simulink model "CACC"  (R2020a)
settings: Solver=VariableStepAuto  StartTime=0.0  StopTime=100  RelTol=1e-3
InitFcn:
  | totalVehicles = 2;
  | if exist('vehStatesBus', 'var')==0
  | load vehBuses
  | end
  | if exist('vehErrorsBus', 'var')==0
  | load vehBuses
  | end
libraries: simulink x9, sim3dlib x2, sim3dautolib x2, autolibshared x2, visionsinks x1
settings Model: Creator=fvall  LastModifiedBy=fvall

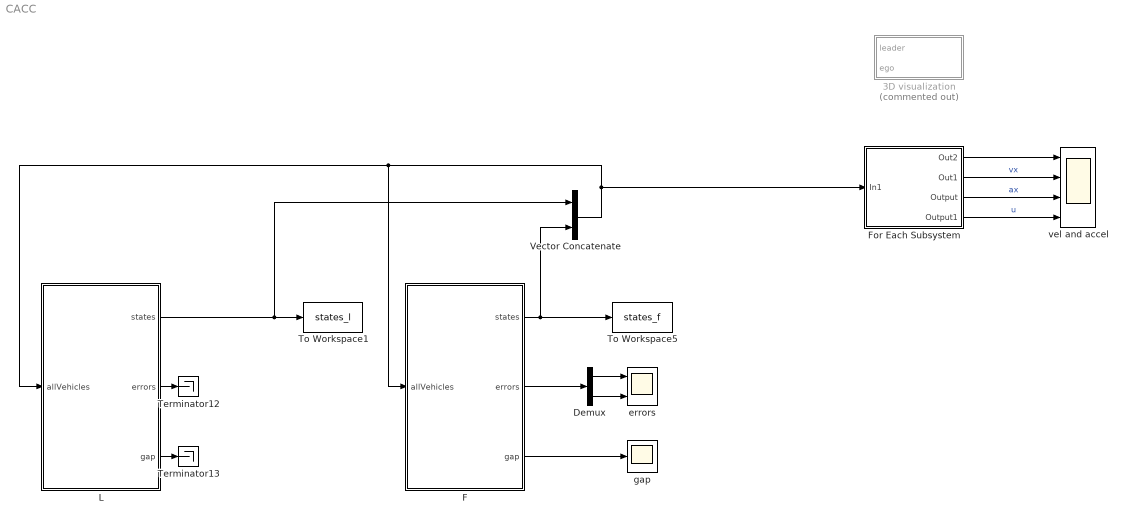
== system CACC ==
  3D visualization : Subsystem  Commented=on
  Demux : Demux  Outputs=2
  F : Subsystem  mask{m=2000, lf=2.5, lr=2.5, maxAcceleration=3, minAcceleration=-8, maxJerk=50, minJerk=-50, freeFlowVel=25, tau=0.5, x0=0, vx0=20, y0=0, h=0.56375, d0=0.32452, minHeadwayError=-100, maxHeadwayError=Inf, velFilterGain=10, Kd=1.7738, Kp=0.17738, Ki=0, Ka=0.97561, Kdd=0.097561, velKi=0.0019848, velKp=0.052702, velKd=-0.65465, hFilterGain=1, hFilterSaturation=0.5, vMin=13, maxComfAccel=0.6, minComfAccel=-0.4, maxComfJerk=10, minComfJerk=-10, hLC=1.6381, d0LC=0.32452}
      mask prompts: m "autoblks_shared:autoblkVehBody3DofLat:blkPrm_m"; lf "autoblks_shared:autoblkVehBody3DofLat:blkPrm_a"; lr "autoblks_shared:autoblkVehBody3DofLat:blkPrm_b"; maxAcceleration "Max Acceleration"; minAcceleration "Min Acceleration"; maxJerk "Max Jerk"; minJerk "Min Jerk"; freeFlowVel "Free Flow Velocity"; tau "Actuator Lag"; x0 "autoblks_shared:autoblkVehBody3DofLat:blkPrm_X_o"; vx0 "autoblks_shared:autoblkVehBody3DofLat:blkPrm_xdot_o"; y0 "autoblks_shared:autoblkVehBody3DofLat:blkPrm_Y_o"; h "Time Headway"; d0 "Standstill Gap"; minHeadwayError "Min Headway Error"; maxHeadwayError "Max Headway Error"; velFilterGain "Velocity Filter Gain"; hFilterGain "Headway Filter Gain"; hFilterSaturation "Headway Filter Saturation"; vMin "Min Velocity"; maxComfAccel "Max Comf Accel"; minComfAccel "Min Comf Accel"; maxComfJerk "Max Comf Jerk"; minComfJerk "Min Comf Jerk"; hLC "Time Headway LC"; d0LC "Standstill Gap LC"
      mask TypeOptions m: Vehicle Body 3DOF Single Track/m
      mask TypeOptions lf: Vehicle Body 3DOF Single Track/a
      mask TypeOptions lr: Vehicle Body 3DOF Single Track/b
      mask TypeOptions x0: Vehicle Body 3DOF Single Track/X_o
      mask TypeOptions vx0: Vehicle Body 3DOF Single Track/xdot_o
      mask TypeOptions y0: Vehicle Body 3DOF Single Track/Y_o
      mask DialogControl DescGroupVar Prompt: 3DOF Vehicle with ACC
      mask DialogControl DescTextVar Prompt: Vehicle with ACC. The vehicle model is Simulink's 3DOF single track vehicle body. The controller is a PID with constant headway including headway error saturation and filtered leader velocity.
      mask DialogControl VehParams Prompt: Vehicle Parameters
      mask DialogControl m Prompt: Vehicle mass, m [kg]:
      mask DialogControl lf Prompt: Longitudinal distance from center of mass to front axle, a [m]:
      mask DialogControl lr Prompt: Longitudinal distance from center of mass to rear axle, b [m]:
      mask DialogControl InitStates Prompt: Initial State
      mask DialogControl x0 Prompt: Initial inertial frame longitudinal position, X_o [m]:
      mask DialogControl vx0 Prompt: Initial longitudinal velocity, xdot_o [m/s]:
      mask DialogControl y0 Prompt: Initial inertial frame lateral displacement, Y_o [m]:
      mask DialogControl Container3 Prompt: Veh Following Parameters
      mask DialogControl ComfortConstraints Prompt: Comfort Constraints
      mask DialogControl LaneChangeParams Prompt: Lane Change Params
  For Each Subsystem : Subsystem  TreatAsAtomicUnit=on
  L : Subsystem  mask{m=2000, lf=2.5, lr=2.5, maxAcceleration=3, minAcceleration=-8, maxJerk=50, minJerk=-50, freeFlowVel=20, tau=0.5, x0=316.5995, vx0=20, y0=0, h=0.56375, d0=0.32452, minHeadwayError=-100, maxHeadwayError=Inf, velFilterGain=10, Kd=1.7738, Kp=0.17738, Ki=0, Ka=0.97561, Kdd=0.097561, velKi=0.0019848, velKp=0.052702, velKd=-0.65465, hFilterGain=1, hFilterSaturation=0.5, vMin=13, maxComfAccel=0.6, minComfAccel=-0.4, maxComfJerk=10, minComfJerk=-10, hLC=1.6381, d0LC=0.32452}
      mask prompts: m "autoblks_shared:autoblkVehBody3DofLat:blkPrm_m"; lf "autoblks_shared:autoblkVehBody3DofLat:blkPrm_a"; lr "autoblks_shared:autoblkVehBody3DofLat:blkPrm_b"; maxAcceleration "Max Acceleration"; minAcceleration "Min Acceleration"; maxJerk "Max Jerk"; minJerk "Min Jerk"; freeFlowVel "Free Flow Velocity"; tau "Actuator Lag"; x0 "autoblks_shared:autoblkVehBody3DofLat:blkPrm_X_o"; vx0 "autoblks_shared:autoblkVehBody3DofLat:blkPrm_xdot_o"; y0 "autoblks_shared:autoblkVehBody3DofLat:blkPrm_Y_o"; h "Time Headway"; d0 "Standstill Gap"; minHeadwayError "Min Headway Error"; maxHeadwayError "Max Headway Error"; velFilterGain "Velocity Filter Gain"; hFilterGain "Headway Filter Gain"; hFilterSaturation "Headway Filter Saturation"; vMin "Min Velocity"; maxComfAccel "Max Comf Accel"; minComfAccel "Min Comf Accel"; maxComfJerk "Max Comf Jerk"; minComfJerk "Min Comf Jerk"; hLC "Time Headway LC"; d0LC "Standstill Gap LC"
      mask TypeOptions m: Vehicle Body 3DOF Single Track/m
      mask TypeOptions lf: Vehicle Body 3DOF Single Track/a
      mask TypeOptions lr: Vehicle Body 3DOF Single Track/b
      mask TypeOptions x0: Vehicle Body 3DOF Single Track/X_o
      mask TypeOptions vx0: Vehicle Body 3DOF Single Track/xdot_o
      mask TypeOptions y0: Vehicle Body 3DOF Single Track/Y_o
      mask DialogControl DescGroupVar Prompt: 3DOF Vehicle with ACC
      mask DialogControl DescTextVar Prompt: Vehicle with ACC. The vehicle model is Simulink's 3DOF single track vehicle body. The controller is a PID with constant headway including headway error saturation and filtered leader velocity.
      mask DialogControl VehParams Prompt: Vehicle Parameters
      mask DialogControl m Prompt: Vehicle mass, m [kg]:
      mask DialogControl lf Prompt: Longitudinal distance from center of mass to front axle, a [m]:
      mask DialogControl lr Prompt: Longitudinal distance from center of mass to rear axle, b [m]:
      mask DialogControl InitStates Prompt: Initial State
      mask DialogControl x0 Prompt: Initial inertial frame longitudinal position, X_o [m]:
      mask DialogControl vx0 Prompt: Initial longitudinal velocity, xdot_o [m/s]:
      mask DialogControl y0 Prompt: Initial inertial frame lateral displacement, Y_o [m]:
      mask DialogControl Container3 Prompt: Veh Following Parameters
      mask DialogControl ComfortConstraints Prompt: Comfort Constraints
      mask DialogControl LaneChangeParams Prompt: Lane Change Params
  Terminator12 : Terminator
  Terminator13 : Terminator
  To Workspace1 : ToWorkspace  VariableName=states_l  SaveFormat=Timeseries  SampleTime=-1
  To Workspace5 : ToWorkspace  VariableName=states_f  SaveFormat=Timeseries  SampleTime=-1
  Vector Concatenate : Concatenate
  errors : Scope  NumInputPorts=2
  gap : Scope
  vel and accel : Scope  NumInputPorts=4
  wires:
  L/1(states) -> Vector Concatenate/1, To Workspace1/1
  F/1(states) -> To Workspace5/1, Vector Concatenate/2
  Vector Concatenate/1 -> F/1(allVehicles), L/1(allVehicles), For Each Subsystem/1(In1)
  F/2(errors) -> Demux/1
  Demux/1 -> errors/1
  Demux/2 -> errors/2
  F/3(gap) -> gap/1
  For Each Subsystem/3(Output) -> vel and accel/3  "ax"
  For Each Subsystem/2(Out1) -> vel and accel/2  "vx"
  L/2(errors) -> Terminator12/1
  L/3(gap) -> Terminator13/1
  For Each Subsystem/4(Output1) -> vel and accel/4  "u"
  For Each Subsystem/1(Out2) -> vel and accel/1

== system CACC/3D visualization ==
  leader : Inport
  ego : Inport  Port=2
  Bus Selector : BusSelector  OutputSignals=InertFrm.Geom.Disp.X,InertFrm.Geom.Disp.Y,InertFrm.Cg.Ang.psi
  Bus Selector1 : BusSelector  OutputSignals=InertFrm.Geom.Disp.X,InertFrm.Geom.Disp.Y,InertFrm.Cg.Ang.psi
  Simulation 3D Camera Get : sim3dlib/Simulation 3D Camera Get  Priority=1  sensorTag=Sim3dSensor1  sensorId=1  sensorName=Sim3dSensor1  vehTagList={'Scene Origin';'SimulinkVehicle1';'SimulinkVehicle2'}  vehTag=SimulinkVehicle1  mountLoc=Rearview mirror  offsetFlag=off  tmountOffset=[0, 0, 0]  rmountOffset=[0, 0, 0]  HorizontalResolution=1280  VerticalResolution=720  HorizontalFOV=60  SampleTime=-1  mountPoint=[0.319999992847443 0 1.19000005722046]  mountOrientation=[0 0 0]  aMode=2  ID=1
      settings: SourceProductBaseCode=DR,VE
  Simulation 3D Scene Configuration : sim3dlib/Simulation 3D Scene Configuration  Priority=0  ProjectFormat=Default Scenes  SceneDesc=Straight road  ProjectName=VehicleSimulation.exe  ScenePath=/Game/Maps/HwStrght  vehTagList={'Scene Origin';'SimulinkVehicle1'}  vehTag=SimulinkVehicle1  OpVisEn=off  Ts=1/60  EnableWindow=on  sensorTag=MainCamera1  sensorId=1  sensorName=MainCamera1  mountLoc=Origin  offsetFlag=off  tmountOffset=[0, 0, 0]  rmountOffset=[0, 0, 0]  HorizontalResolution=1280  VerticalResolution=720  HorizontalFOV=60  mountPoint=[0 0 0]  mountOrientation=[0 0 0]  aMode=3  ID=1
      settings: SourceProductBaseCode=DR,VE
  Simulation 3D Vehicle with Ground Following : sim3dautolib/Simulation 3D Vehicle with Ground Following  Priority=-1  PassVehMesh=Muscle car  VehColor=Red  InitialPos=[0, 0, 0]  InitialRot=[0, 0, 0]  ActorName=SimulinkVehicle1  SampleTime=-1  ActorType=SimulinkVehicle  ID=1  aMode=3  ActorTag=SimulinkVehicle1  CoordinateScheme=ISO  TransformOutportEnabled=off
      settings: SourceProductBaseCode=DR,VE
  Simulation 3D Vehicle with Ground Following1 : sim3dautolib/Simulation 3D Vehicle with Ground Following  Priority=-1  PassVehMesh=Muscle car  VehColor=Red  InitialPos=[0, 0, 0]  InitialRot=[0, 0, 0]  ActorName=SimulinkVehicle2  SampleTime=-1  ActorType=SimulinkVehicle  ID=2  aMode=3  ActorTag=SimulinkVehicle2  CoordinateScheme=ISO  TransformOutportEnabled=off
      settings: SourceProductBaseCode=DR,VE
  Unit Conversion : UnitConversion
  Unit Conversion1 : UnitConversion
  Video To Workspace : visionsinks/Video To Workspace  VariableName=vout  NumInputs=1  DataLimit=1000  DecimationFactor=1  LogFi=off  InPortLabels=R|G|B
      settings: SourceProductBaseCode=VP
  wires:
  Unit Conversion/1 -> Simulation 3D Vehicle with Ground Following/3
  ego/1 -> Bus Selector/1
  Bus Selector/1 -> Simulation 3D Vehicle with Ground Following/1  "<X>"
  Bus Selector/2 -> Simulation 3D Vehicle with Ground Following/2  "<Y>"
  Bus Selector/3 -> Unit Conversion/1  "<psi>"
  Unit Conversion1/1 -> Simulation 3D Vehicle with Ground Following1/3
  leader/1 -> Bus Selector1/1
  Bus Selector1/1 -> Simulation 3D Vehicle with Ground Following1/1  "<X>"
  Bus Selector1/2 -> Simulation 3D Vehicle with Ground Following1/2  "<Y>"
  Bus Selector1/3 -> Unit Conversion1/1  "<psi>"
  Simulation 3D Camera Get/1 -> Video To Workspace/1

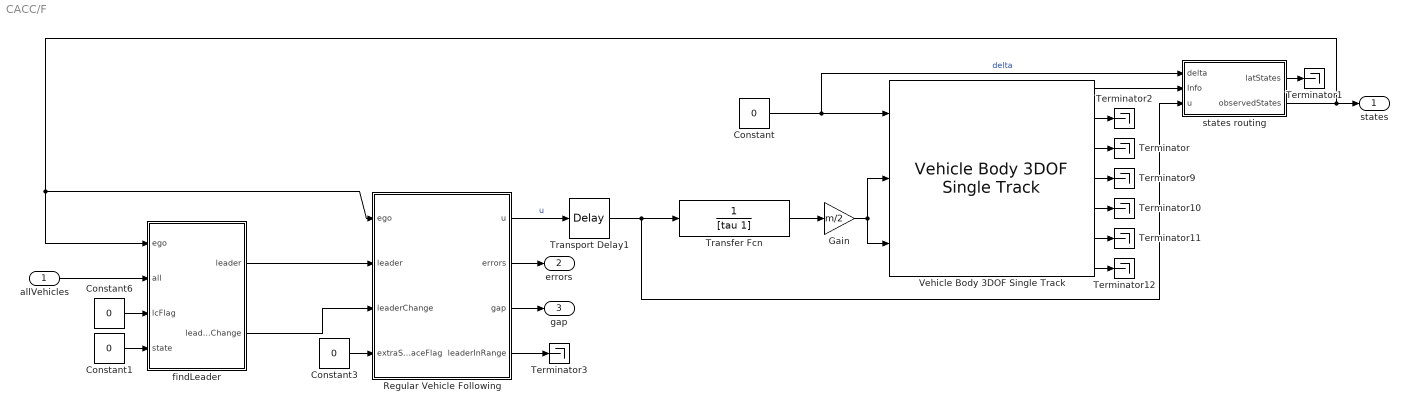
== system CACC/F ==
  allVehicles : Inport
  Constant{,1,3,6} (4 alike) : Constant  Value=0
  Gain : Gain  Gain=m/2
  Regular Vehicle Following : Subsystem
  Terminator{,1..3,9..12} (8 alike) : Terminator
  Transfer Fcn : TransferFcn  Denominator=[tau 1]
  Transport Delay1 : TransportDelay  DelayTime=0.01
  Vehicle Body 3DOF Single Track : autolibshared/Vehicle Body 3DOF Single Track  trackMode=Single (bicycle)  inputMode=External longitudinal forces  frontSteerMode=on  rearSteerMode=off  windMode=off  muMode=off  extFMode=off  extMMode=off  extXo=off  extpsio=off  extxdoto=off  extro=off  extYo=off  extTamb=off  extydoto=off  aMode=2  NF=2  NR=2  m=m  a=lf  b=lr  h=0.35  X_o=x0  xdot_o=vx0  CalphaMode=off  sigmaMode=on  d=0  w=[1.4,1.4]  Cy_f=12e3  Cy_r=11e3  sigma_f=.1  sigma_r=.1  alpha_f_brk=[-.1 .1]  Cy_f_data=[-9e3 9e3]  alpha_r_brk=[-.1 .1]  Cy_r_data=[-9e3 9e3]  Y_o=y0  ydot_o=0  Izz=4000  psi_o=0  r_o=0  Af=2  Cd=.3  Cl=.1  Cpm=.1  beta_w=[0:0.01:0.3]  Cs=[0:0.03:0.9]  Cym=[0:0.01:0.3]  Pabs=101325  Tair=273  g=9.81  mu=1  xdot_tol=.01  Fznom=5000  Fxtire_sat=7e4  Fytire_sat=7e4  longOff=0  latOff=0  vertOff=0  wrapAng=off
      settings: SourceProductBaseCode=PW,MT,VE,VP
  findLeader : Subsystem
  states routing : Subsystem
  states : Outport  VectorParamsAs1DForOutWhenUnconnected=off
  errors : Outport  Port=2  VectorParamsAs1DForOutWhenUnconnected=off
  gap : Outport  Port=3  VectorParamsAs1DForOutWhenUnconnected=off
  wires:
  Transfer Fcn/1 -> Gain/1
  findLeader/1(leader) -> Regular Vehicle Following/2(leader)
  Regular Vehicle Following/4(leaderInRange) -> Terminator3/1
  Constant3/1 -> Regular Vehicle Following/4(extraSpaceFlag)
  Constant/1 -> states routing/1(delta), Vehicle Body 3DOF Single Track/1  "delta"
  Regular Vehicle Following/2(errors) -> errors/1
  Regular Vehicle Following/1(u) -> Transport Delay1/1  "u"
  findLeader/2(leaderChange) -> Regular Vehicle Following/3(leaderChange)
  Transport Delay1/1 -> states routing/3(u), Transfer Fcn/1
  states routing/2(observedStates) -> Regular Vehicle Following/1(ego), findLeader/1(ego), states/1
  Vehicle Body 3DOF Single Track/1 -> states routing/2(Info)
  Gain/1 -> Vehicle Body 3DOF Single Track/3, Vehicle Body 3DOF Single Track/2
  allVehicles/1 -> findLeader/2(all)
  Regular Vehicle Following/3(gap) -> gap/1
  Constant1/1 -> findLeader/4(state)
  Constant6/1 -> findLeader/3(lcFlag)
  states routing/1(latStates) -> Terminator1/1
  Vehicle Body 3DOF Single Track/2 -> Terminator2/1
  Vehicle Body 3DOF Single Track/5 -> Terminator10/1
  Vehicle Body 3DOF Single Track/3 -> Terminator/1
  Vehicle Body 3DOF Single Track/6 -> Terminator11/1
  Vehicle Body 3DOF Single Track/7 -> Terminator12/1
  Vehicle Body 3DOF Single Track/4 -> Terminator9/1

== system CACC/For Each Subsystem ==
  In1 : Inport  Partition=on  PartitionDimension=1  PartitionWidth=1  PartitionOffset=0
  Bus Selector : BusSelector  OutputSignals=X,Xdot,xddot,u
  For Each : ForEach  DisableCoverage=on
  Out2 : Outport  ConcatenationDimension=1
  Out1 : Outport  Port=2  ConcatenationDimension=1
  Output : Outport  Port=3  ConcatenationDimension=1
  Output1 : Outport  Port=4  ConcatenationDimension=1
  wires:
  In1/1 -> Bus Selector/1
  Bus Selector/2 -> Out1/1  "<Xdot>"
  Bus Selector/3 -> Output/1  "<xddot>"
  Bus Selector/4 -> Output1/1  "<u>"
  Bus Selector/1 -> Out2/1  "<X>"

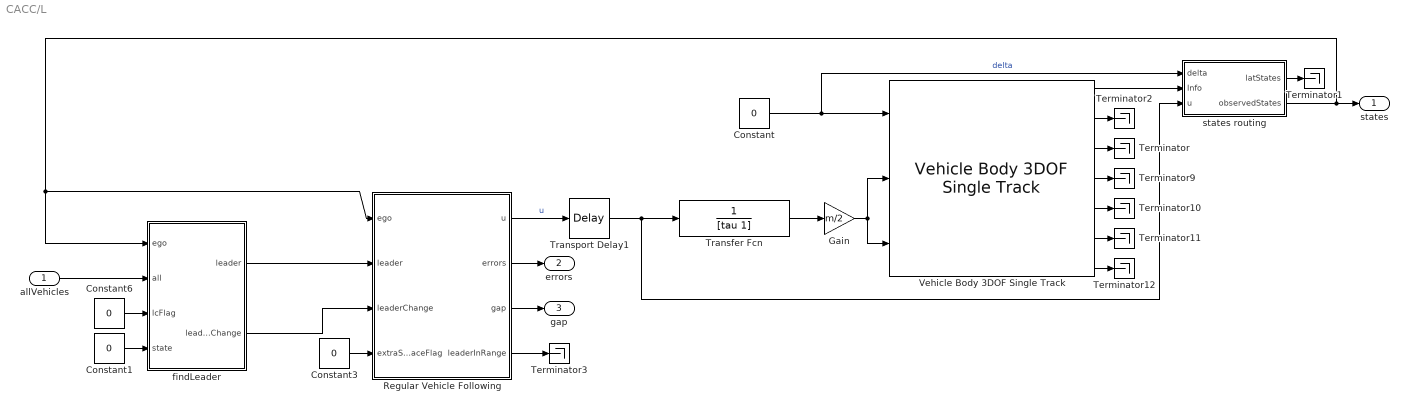
== system CACC/L ==
  allVehicles : Inport
  Constant{,1,3,6} (4 alike) : Constant  Value=0
  Gain : Gain  Gain=m/2
  Regular Vehicle Following : Subsystem
  Terminator{,1..3,9..12} (8 alike) : Terminator
  Transfer Fcn : TransferFcn  Denominator=[tau 1]
  Transport Delay1 : TransportDelay  DelayTime=0.01
  Vehicle Body 3DOF Single Track : autolibshared/Vehicle Body 3DOF Single Track  trackMode=Single (bicycle)  inputMode=External longitudinal forces  frontSteerMode=on  rearSteerMode=off  windMode=off  muMode=off  extFMode=off  extMMode=off  extXo=off  extpsio=off  extxdoto=off  extro=off  extYo=off  extTamb=off  extydoto=off  aMode=2  NF=2  NR=2  m=m  a=lf  b=lr  h=0.35  X_o=x0  xdot_o=vx0  CalphaMode=off  sigmaMode=on  d=0  w=[1.4,1.4]  Cy_f=12e3  Cy_r=11e3  sigma_f=.1  sigma_r=.1  alpha_f_brk=[-.1 .1]  Cy_f_data=[-9e3 9e3]  alpha_r_brk=[-.1 .1]  Cy_r_data=[-9e3 9e3]  Y_o=y0  ydot_o=0  Izz=4000  psi_o=0  r_o=0  Af=2  Cd=.3  Cl=.1  Cpm=.1  beta_w=[0:0.01:0.3]  Cs=[0:0.03:0.9]  Cym=[0:0.01:0.3]  Pabs=101325  Tair=273  g=9.81  mu=1  xdot_tol=.01  Fznom=5000  Fxtire_sat=7e4  Fytire_sat=7e4  longOff=0  latOff=0  vertOff=0  wrapAng=off
      settings: SourceProductBaseCode=PW,MT,VE,VP
  findLeader : Subsystem
  states routing : Subsystem
  states : Outport  VectorParamsAs1DForOutWhenUnconnected=off
  errors : Outport  Port=2  VectorParamsAs1DForOutWhenUnconnected=off
  gap : Outport  Port=3  VectorParamsAs1DForOutWhenUnconnected=off
  wires:
  Transfer Fcn/1 -> Gain/1
  findLeader/1(leader) -> Regular Vehicle Following/2(leader)
  Regular Vehicle Following/4(leaderInRange) -> Terminator3/1
  Constant3/1 -> Regular Vehicle Following/4(extraSpaceFlag)
  Constant/1 -> states routing/1(delta), Vehicle Body 3DOF Single Track/1  "delta"
  Regular Vehicle Following/2(errors) -> errors/1
  Regular Vehicle Following/1(u) -> Transport Delay1/1  "u"
  findLeader/2(leaderChange) -> Regular Vehicle Following/3(leaderChange)
  Transport Delay1/1 -> states routing/3(u), Transfer Fcn/1
  states routing/2(observedStates) -> Regular Vehicle Following/1(ego), findLeader/1(ego), states/1
  Vehicle Body 3DOF Single Track/1 -> states routing/2(Info)
  Gain/1 -> Vehicle Body 3DOF Single Track/3, Vehicle Body 3DOF Single Track/2
  allVehicles/1 -> findLeader/2(all)
  Regular Vehicle Following/3(gap) -> gap/1
  Constant1/1 -> findLeader/4(state)
  Constant6/1 -> findLeader/3(lcFlag)
  states routing/1(latStates) -> Terminator1/1
  Vehicle Body 3DOF Single Track/2 -> Terminator2/1
  Vehicle Body 3DOF Single Track/5 -> Terminator10/1
  Vehicle Body 3DOF Single Track/3 -> Terminator/1
  Vehicle Body 3DOF Single Track/6 -> Terminator11/1
  Vehicle Body 3DOF Single Track/7 -> Terminator12/1
  Vehicle Body 3DOF Single Track/4 -> Terminator9/1

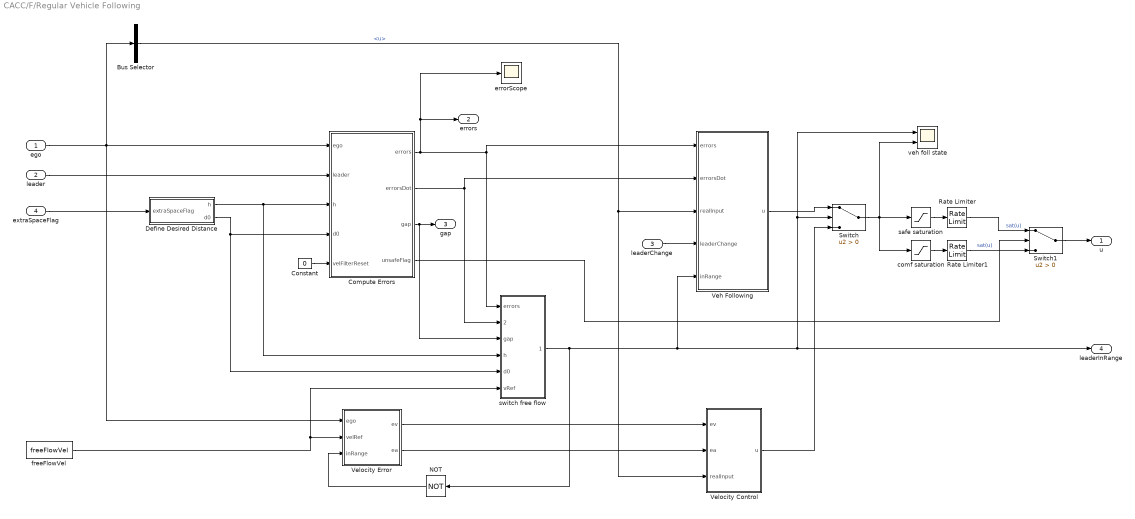
== system CACC/F/Regular Vehicle Following ==
  ego : Inport
  leader : Inport  Port=2
  leaderChange : Inport  Port=3
  extraSpaceFlag : Inport  Port=4
  Bus Selector : BusSelector  OutputSignals=u
  Compute Errors : Subsystem
  Constant : Constant  Value=0
  Define Desired Distance : Subsystem
  NOT : Logic  Operator=NOT  IconShape=distinctive  AllPortsSameDT=off  OutDataTypeStr=boolean
  Rate Limiter : RateLimiter  RisingSlewLimit=maxJerk  FallingSlewLimit=minJerk  SampleTimeMode=inherited
  Rate Limiter1 : RateLimiter  RisingSlewLimit=maxComfJerk  FallingSlewLimit=minComfJerk  SampleTimeMode=inherited
  Switch : Switch  Criteria=u2 > Threshold
  Switch1 : Switch  Criteria=u2 > Threshold
  Veh Following : Subsystem  TreatAsAtomicUnit=on
  Velocity Control : Subsystem  TreatAsAtomicUnit=on
  Velocity Error : Subsystem
  comf saturation : Saturate  UpperLimit=maxComfAccel  LowerLimit=minComfAccel
  errorScope : Scope
  freeFlowVel : Constant  Value=freeFlowVel
  safe saturation : Saturate  UpperLimit=maxAcceleration  LowerLimit=minAcceleration
  switch free flow : Subsystem
  veh foll state : Scope  NumInputPorts=2
  u : Outport  VectorParamsAs1DForOutWhenUnconnected=off
  errors : Outport  Port=2  VectorParamsAs1DForOutWhenUnconnected=off
  gap : Outport  Port=3  VectorParamsAs1DForOutWhenUnconnected=off
  leaderInRange : Outport  Port=4  VectorParamsAs1DForOutWhenUnconnected=off
  wires:
  Define Desired Distance/2(d0) -> switch free flow/5(d0), Compute Errors/4(d0)
  Define Desired Distance/1(h) -> switch free flow/4(h), Compute Errors/3(h)
  extraSpaceFlag/1 -> Define Desired Distance/1(extraSpaceFlag)
  Compute Errors/2(errorsDot) -> switch free flow/2(errorsDot), Veh Following/2(errorsDot)
  Bus Selector/1 -> Velocity Control/3(realInput), Veh Following/3(realInput)  "<u>"
  Compute Errors/4(unsafeFlag) -> Switch1/2
  freeFlowVel/1 -> switch free flow/6(vRef), Velocity Error/2(velRef)
  Velocity Control/1(u) -> Switch/3
  ego/1 -> Velocity Error/1(ego), Bus Selector/1, Compute Errors/1(ego)
  Compute Errors/3("gap ") -> switch free flow/3(gap), gap/1
  Rate Limiter1/1 -> Switch1/3  "sat(u)"
  Switch/1 -> comf saturation/1, safe saturation/1, veh foll state/2
  Switch1/1 -> u/1
  Rate Limiter/1 -> Switch1/1  "sat(u)"
  safe saturation/1 -> Rate Limiter/1
  comf saturation/1 -> Rate Limiter1/1
  Compute Errors/1(errors) -> errorScope/1, errors/1, switch free flow/1(errors), Veh Following/1(errors)
  switch free flow/1(inRange) -> NOT/1, Veh Following/5(inRange), leaderInRange/1, Switch/2, veh foll state/1
  leader/1 -> Compute Errors/2(leader)
  Constant/1 -> Compute Errors/5(velFilterReset)
  Veh Following/1(u) -> Switch/1
  leaderChange/1 -> Veh Following/4(leaderChange)
  Velocity Error/2(ea) -> Velocity Control/2(ea)
  Velocity Error/1(ev) -> Velocity Control/1(ev)
  NOT/1 -> Velocity Error/3(inRange)

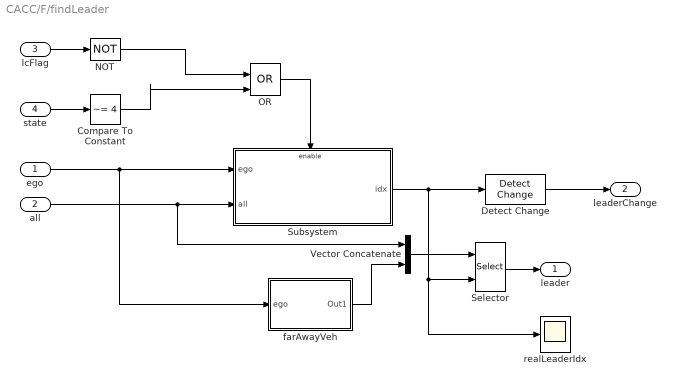
== system CACC/F/findLeader ==
  ego : Inport
  all : Inport  Port=2
  lcFlag : Inport  Port=3
  state : Inport  Port=4
  Compare To Constant : simulink/Logic and Bit Operations/Compare To Constant  relop=~=  const=4  OutDataTypeStr=boolean
  Detect Change : simulink/Logic and Bit Operations/Detect Change  vinit=0  OutDataTypeStr=boolean
  NOT : Logic  Operator=NOT  IconShape=distinctive  AllPortsSameDT=off  OutDataTypeStr=boolean
  OR : Logic  Operator=OR  IconShape=distinctive  AllPortsSameDT=off  OutDataTypeStr=boolean
  Selector : Selector  InputPortWidth=totalVehicles+1  IndexOptions=Index vector (port)  Indices=[1]  OutputSizes=1
  Subsystem : Subsystem
  Vector Concatenate : Concatenate
  farAwayVeh : Subsystem
  realLeaderIdx : Scope
  leader : Outport  VectorParamsAs1DForOutWhenUnconnected=off
  leaderChange : Outport  Port=2  InitialOutput=1  VectorParamsAs1DForOutWhenUnconnected=off
  wires:
  Detect Change/1 -> leaderChange/1
  Vector Concatenate/1 -> Selector/1
  farAwayVeh/1(Out1) -> Vector Concatenate/2
  Selector/1 -> leader/1
  NOT/1 -> OR/1
  lcFlag/1 -> NOT/1
  OR/1 -> Subsystem/Enable
  Subsystem/1(idx) -> Detect Change/1, Selector/2, realLeaderIdx/1
  all/1 -> Subsystem/2(all), Vector Concatenate/1
  ego/1 -> Subsystem/1(ego), farAwayVeh/1(ego)
  state/1 -> Compare To Constant/1
  Compare To Constant/1 -> OR/2

== system CACC/F/states routing ==
  delta : Inport
  Info : Inport  Port=2
  u : Inport  Port=3
  Bus Creator : BusCreator  Inputs=7  OutDataTypeStr=Bus: vehStatesBus  NonVirtualBus=on
      settings: InheritFromInputs=off
  Bus Selector : BusSelector  OutputSignals=BdyFrm.Cg.Vel.ydot,BdyFrm.Cg.AngVel.r,InertFrm.RearAxl.Disp.X,InertFrm.Cg.Disp.Y,InertFrm.RearAxl.Vel.Xdot,BdyFrm.Cg.Acc.xddot,InertFrm.Cg.Ang.psi
  Mux : Mux
  latStates : Outport
  observedStates : Outport  Port=2
  wires:
  Info/1 -> Bus Selector/1
  Bus Selector/3 -> Bus Creator/1  "<X>"
  Bus Selector/4 -> Bus Creator/2, Mux/1  "<Y>"
  Bus Selector/5 -> Bus Creator/3  "<Xdot>"
  Bus Selector/6 -> Bus Creator/4  "<xddot>"
  Bus Selector/7 -> Bus Creator/5, Mux/3  "<psi>"
  u/1 -> Bus Creator/6  "u"
  delta/1 -> Bus Creator/7
  Mux/1 -> latStates/1
  Bus Selector/1 -> Mux/2  "<ydot>"
  Bus Selector/2 -> Mux/4  "<r>"
  Bus Creator/1 -> observedStates/1

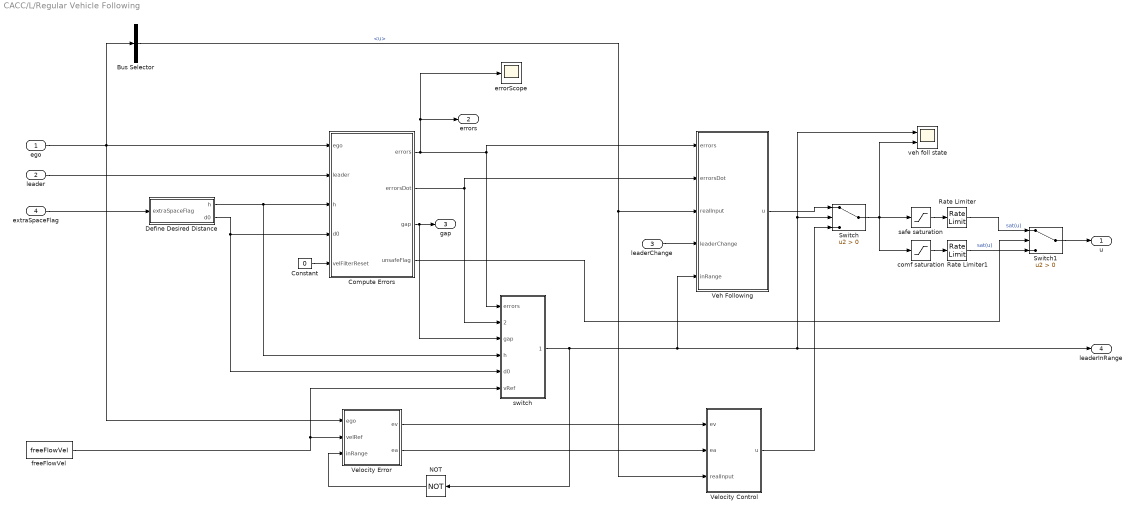
== system CACC/L/Regular Vehicle Following ==
  ego : Inport
  leader : Inport  Port=2
  leaderChange : Inport  Port=3
  extraSpaceFlag : Inport  Port=4
  Bus Selector : BusSelector  OutputSignals=u
  Compute Errors : Subsystem
  Constant : Constant  Value=0
  Define Desired Distance : Subsystem
  NOT : Logic  Operator=NOT  IconShape=distinctive  AllPortsSameDT=off  OutDataTypeStr=boolean
  Rate Limiter : RateLimiter  RisingSlewLimit=maxJerk  FallingSlewLimit=minJerk  SampleTimeMode=inherited
  Rate Limiter1 : RateLimiter  RisingSlewLimit=maxComfJerk  FallingSlewLimit=minComfJerk  SampleTimeMode=inherited
  Switch : Switch  Criteria=u2 > Threshold
  Switch1 : Switch  Criteria=u2 > Threshold
  Veh Following : Subsystem  TreatAsAtomicUnit=on
  Velocity Control : Subsystem  TreatAsAtomicUnit=on
  Velocity Error : Subsystem
  comf saturation : Saturate  UpperLimit=maxComfAccel  LowerLimit=minComfAccel
  errorScope : Scope
  freeFlowVel : Constant  Value=freeFlowVel
  safe saturation : Saturate  UpperLimit=maxAcceleration  LowerLimit=minAcceleration
  switch : Subsystem
  veh foll state : Scope  NumInputPorts=2
  u : Outport  VectorParamsAs1DForOutWhenUnconnected=off
  errors : Outport  Port=2  VectorParamsAs1DForOutWhenUnconnected=off
  gap : Outport  Port=3  VectorParamsAs1DForOutWhenUnconnected=off
  leaderInRange : Outport  Port=4  VectorParamsAs1DForOutWhenUnconnected=off
  wires:
  Define Desired Distance/2(d0) -> switch/5(d0), Compute Errors/4(d0)
  Define Desired Distance/1(h) -> switch/4(h), Compute Errors/3(h)
  extraSpaceFlag/1 -> Define Desired Distance/1(extraSpaceFlag)
  Compute Errors/2(errorsDot) -> Veh Following/2(errorsDot), switch/2(errorsDot)
  Bus Selector/1 -> Velocity Control/3(realInput), Veh Following/3(realInput)  "<u>"
  Compute Errors/4(unsafeFlag) -> Switch1/2
  freeFlowVel/1 -> switch/6(vRef), Velocity Error/2(velRef)
  Velocity Control/1(u) -> Switch/3
  ego/1 -> Velocity Error/1(ego), Bus Selector/1, Compute Errors/1(ego)
  Compute Errors/3("gap ") -> switch/3(gap), gap/1
  Rate Limiter1/1 -> Switch1/3  "sat(u)"
  Switch/1 -> comf saturation/1, safe saturation/1, veh foll state/2
  Switch1/1 -> u/1
  Rate Limiter/1 -> Switch1/1  "sat(u)"
  safe saturation/1 -> Rate Limiter/1
  comf saturation/1 -> Rate Limiter1/1
  Compute Errors/1(errors) -> errorScope/1, errors/1, Veh Following/1(errors), switch/1(errors)
  switch/1(inRange) -> NOT/1, Veh Following/5(inRange), leaderInRange/1, Switch/2, veh foll state/1
  leader/1 -> Compute Errors/2(leader)
  Constant/1 -> Compute Errors/5(velFilterReset)
  Veh Following/1(u) -> Switch/1
  leaderChange/1 -> Veh Following/4(leaderChange)
  Velocity Error/2(ea) -> Velocity Control/2(ea)
  Velocity Error/1(ev) -> Velocity Control/1(ev)
  NOT/1 -> Velocity Error/3(inRange)

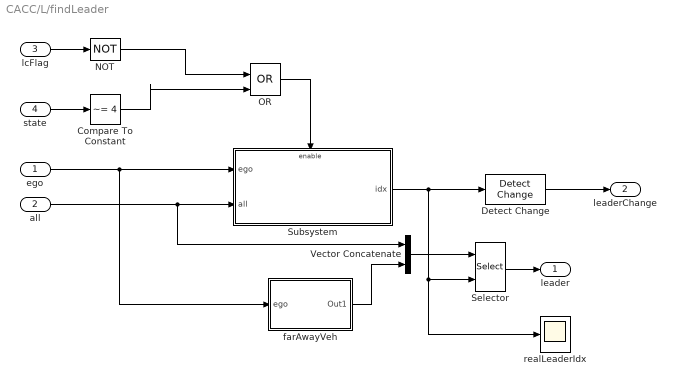
== system CACC/L/findLeader ==
  ego : Inport
  all : Inport  Port=2
  lcFlag : Inport  Port=3
  state : Inport  Port=4
  Compare To Constant : simulink/Logic and Bit Operations/Compare To Constant  relop=~=  const=4  OutDataTypeStr=boolean
  Detect Change : simulink/Logic and Bit Operations/Detect Change  vinit=0  OutDataTypeStr=boolean
  NOT : Logic  Operator=NOT  IconShape=distinctive  AllPortsSameDT=off  OutDataTypeStr=boolean
  OR : Logic  Operator=OR  IconShape=distinctive  AllPortsSameDT=off  OutDataTypeStr=boolean
  Selector : Selector  InputPortWidth=totalVehicles+1  IndexOptions=Index vector (port)  Indices=[1]  OutputSizes=1
  Subsystem : Subsystem
  Vector Concatenate : Concatenate
  farAwayVeh : Subsystem
  realLeaderIdx : Scope
  leader : Outport  VectorParamsAs1DForOutWhenUnconnected=off
  leaderChange : Outport  Port=2  InitialOutput=1  VectorParamsAs1DForOutWhenUnconnected=off
  wires:
  Detect Change/1 -> leaderChange/1
  Vector Concatenate/1 -> Selector/1
  farAwayVeh/1(Out1) -> Vector Concatenate/2
  Selector/1 -> leader/1
  NOT/1 -> OR/1
  lcFlag/1 -> NOT/1
  OR/1 -> Subsystem/Enable
  Subsystem/1(idx) -> Detect Change/1, Selector/2, realLeaderIdx/1
  all/1 -> Subsystem/2(all), Vector Concatenate/1
  ego/1 -> Subsystem/1(ego), farAwayVeh/1(ego)
  state/1 -> Compare To Constant/1
  Compare To Constant/1 -> OR/2

== system CACC/L/states routing ==
  delta : Inport
  Info : Inport  Port=2
  u : Inport  Port=3
  Bus Creator : BusCreator  Inputs=7  OutDataTypeStr=Bus: vehStatesBus  NonVirtualBus=on
      settings: InheritFromInputs=off
  Bus Selector : BusSelector  OutputSignals=BdyFrm.Cg.Vel.ydot,BdyFrm.Cg.AngVel.r,InertFrm.RearAxl.Disp.X,InertFrm.Cg.Disp.Y,InertFrm.RearAxl.Vel.Xdot,BdyFrm.Cg.Acc.xddot,InertFrm.Cg.Ang.psi
  Mux : Mux
  latStates : Outport
  observedStates : Outport  Port=2
  wires:
  Info/1 -> Bus Selector/1
  Bus Selector/3 -> Bus Creator/1  "<X>"
  Bus Selector/4 -> Bus Creator/2, Mux/1  "<Y>"
  Bus Selector/5 -> Bus Creator/3  "<Xdot>"
  Bus Selector/6 -> Bus Creator/4  "<xddot>"
  Bus Selector/7 -> Bus Creator/5, Mux/3  "<psi>"
  u/1 -> Bus Creator/6  "u"
  delta/1 -> Bus Creator/7
  Mux/1 -> latStates/1
  Bus Selector/1 -> Mux/2  "<ydot>"
  Bus Selector/2 -> Mux/4  "<r>"
  Bus Creator/1 -> observedStates/1

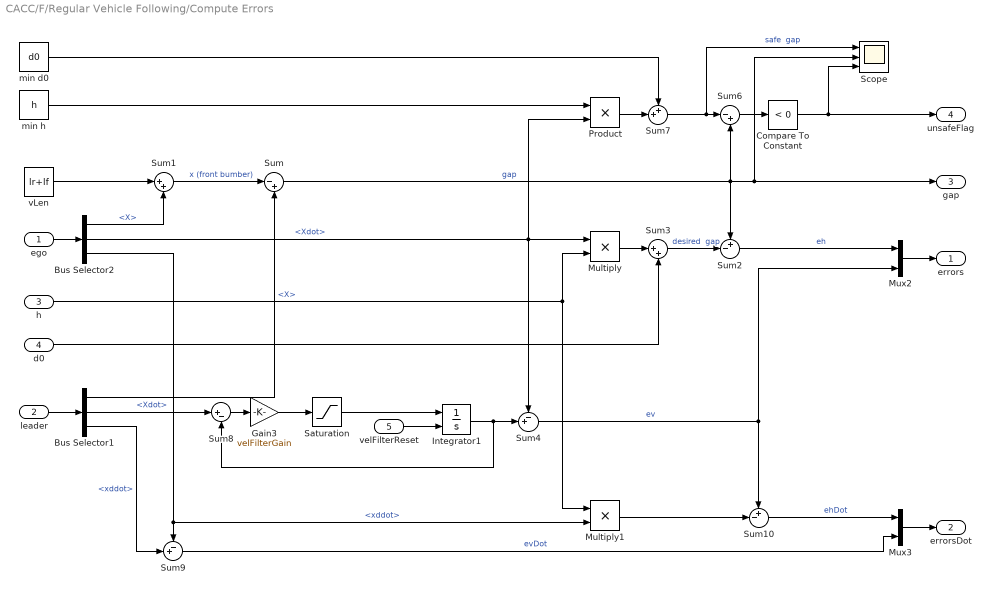
== system CACC/F/Regular Vehicle Following/Compute Errors ==
  ego : Inport
  leader : Inport  Port=2
  h : Inport  Port=3
  d0 : Inport  Port=4
  velFilterReset : Inport  Port=5
  Bus Selector1 : BusSelector  OutputSignals=X,Xdot,xddot
  Bus Selector2 : BusSelector  OutputSignals=X,Xdot,xddot
  Compare To Constant : simulink/Logic and Bit Operations/Compare To Constant  relop=<  const=0  OutDataTypeStr=boolean
  Gain3 : Gain  Gain=velFilterGain
  Integrator1 : Integrator  ExternalReset=rising  InitialCondition=vx0
  Multiply : Product
  Multiply1 : Product
  Mux2 : Mux  Inputs=2
  Mux3 : Mux  Inputs=2
  Product : Product
  Saturation : Saturate  UpperLimit=maxAcceleration  LowerLimit=minAcceleration
  Scope : Scope  NumInputPorts=3
  Sum : Sum  Inputs=|-+
  Sum1 : Sum  Inputs=|++
  Sum10 : Sum  Inputs=+-|
  Sum2 : Sum  Inputs=+-|
  Sum3 : Sum  Inputs=|++
  Sum4 : Sum  Inputs=-+|
  Sum6 : Sum  Inputs=|-+
  Sum7 : Sum  Inputs=++|
  Sum8 : Sum  Inputs=|+-
  Sum9 : Sum  Inputs=-+|
  min d0 : Constant  Value=d0
  min h : Constant  Value=h
  vLen : Constant  Value=lr+lf
  errors : Outport  VectorParamsAs1DForOutWhenUnconnected=off
  errorsDot : Outport  Port=2
  "gap " : Outport  Port=3  VectorParamsAs1DForOutWhenUnconnected=off
  unsafeFlag : Outport  Port=4  VectorParamsAs1DForOutWhenUnconnected=off
  wires:
  leader/1 -> Bus Selector1/1
  ego/1 -> Bus Selector2/1
  Mux3/1 -> errorsDot/1
  Sum9/1 -> Mux3/2  "evDot"
  Sum10/1 -> Mux3/1  "ehDot"
  Multiply1/1 -> Sum10/2
  Bus Selector2/3 -> Multiply1/2, Sum9/1  "<xddot>"
  Bus Selector1/3 -> Sum9/2  "<xddot>"
  Sum8/1 -> Gain3/1
  Integrator1/1 -> Sum8/2, Sum4/2
  Saturation/1 -> Integrator1/1
  Gain3/1 -> Saturation/1
  Sum4/1 -> Sum10/1, Mux2/2  "ev"
  Bus Selector1/2 -> Sum8/1  "<Xdot>"
  h/1 -> Multiply1/1, Multiply/2
  Bus Selector2/1 -> Sum1/2  "<X>"
  Sum/1 -> "gap "/1, Scope/2, Sum6/2, Sum2/1  "gap"
  Multiply/1 -> Sum3/1
  min d0/1 -> Sum7/1
  vLen/1 -> Sum1/1
  d0/1 -> Sum3/2
  Bus Selector2/2 -> Product/2, Multiply/1, Sum4/1  "<Xdot>"
  Sum1/1 -> Sum/1  "x (front bumber)"
  Sum3/1 -> Sum2/2  "desired  gap"
  Product/1 -> Sum7/2
  Bus Selector1/1 -> Sum/2  "<X>"
  Sum2/1 -> Mux2/1  "eh"
  Compare To Constant/1 -> Scope/3, unsafeFlag/1
  min h/1 -> Product/1
  Sum7/1 -> Scope/1, Sum6/1  "safe  gap"
  Sum6/1 -> Compare To Constant/1
  velFilterReset/1 -> Integrator1/2
  Mux2/1 -> errors/1

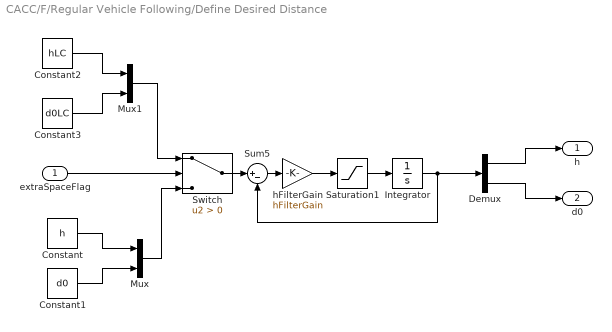
== system CACC/F/Regular Vehicle Following/Define Desired Distance ==
  extraSpaceFlag : Inport
  Constant : Constant  Value=h
  Constant1 : Constant  Value=d0
  Constant2 : Constant  Value=hLC
  Constant3 : Constant  Value=d0LC
  Demux : Demux  Outputs=2
  Integrator : Integrator  InitialCondition=[h d0]
  Mux : Mux  Inputs=2
  Mux1 : Mux  Inputs=2
  Saturation1 : Saturate  UpperLimit=hFilterSaturation  LowerLimit=-hFilterSaturation
  Sum5 : Sum  Inputs=|+-
  Switch : Switch  Criteria=u2 > Threshold
  hFilterGain : Gain  Gain=hFilterGain
  h : Outport
  d0 : Outport  Port=2
  wires:
  Demux/2 -> d0/1
  Demux/1 -> h/1
  Integrator/1 -> Sum5/2, Demux/1
  Saturation1/1 -> Integrator/1
  extraSpaceFlag/1 -> Switch/2
  Constant1/1 -> Mux/2
  Constant3/1 -> Mux1/2
  Switch/1 -> Sum5/1
  Mux1/1 -> Switch/1
  Sum5/1 -> hFilterGain/1
  Constant2/1 -> Mux1/1
  hFilterGain/1 -> Saturation1/1
  Constant/1 -> Mux/1
  Mux/1 -> Switch/3

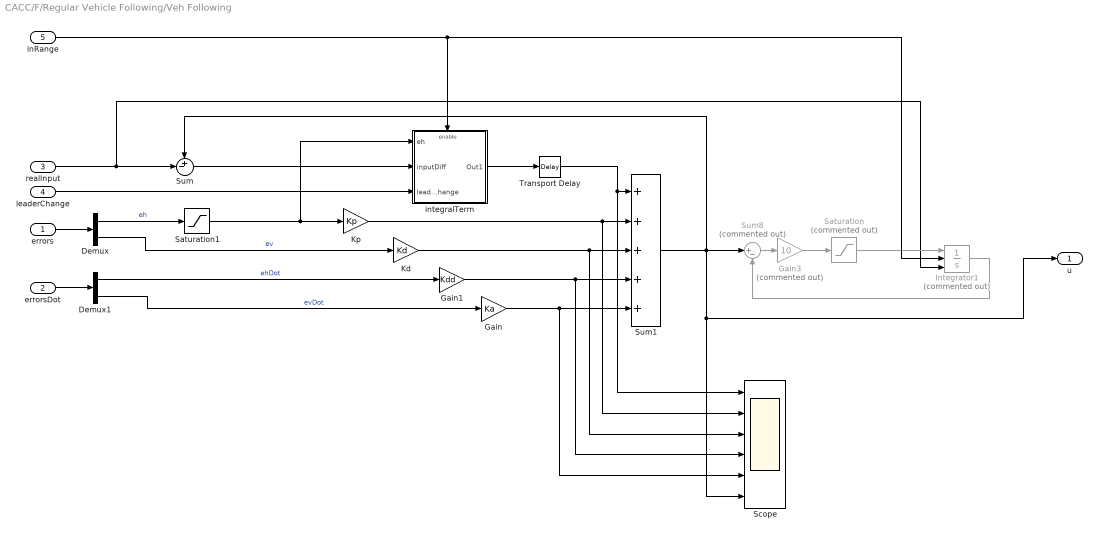
== system CACC/F/Regular Vehicle Following/Veh Following ==
  errors : Inport
  errorsDot : Inport  Port=2
  realInput : Inport  Port=3
  leaderChange : Inport  Port=4
  inRange : Inport  Port=5
  Demux : Demux  Outputs=2
  Demux1 : Demux  Outputs=2
  Gain : Gain  Gain=Ka
  Gain1 : Gain  Gain=Kdd
  Gain3 : Gain  Commented=on  Gain=10
  Integrator1 : Integrator  Commented=on  ExternalReset=rising  InitialConditionSource=external  InitialCondition=vx0
  Kd : Gain  Gain=Kd
  Kp : Gain  Gain=Kp
  Saturation : Saturate  Commented=on  UpperLimit=maxComfAccel  LowerLimit=minAcceleration
  Saturation1 : Saturate  UpperLimit=maxHeadwayError  LowerLimit=minHeadwayError
  Scope : Scope  NumInputPorts=6
  Sum : Sum  Inputs=+-|
  Sum1 : Sum  Inputs=+++++
  Sum8 : Sum  Commented=on  Inputs=|+-
  Transport Delay : TransportDelay  DelayTime=0.1
  integralTerm : Subsystem
  u : Outport  VectorParamsAs1DForOutWhenUnconnected=off
  wires:
  Demux1/2 -> Gain/1  "evDot"
  Demux1/1 -> Gain1/1  "ehDot"
  errorsDot/1 -> Demux1/1
  Sum1/1 -> Scope/6, u/1, Sum/1, Sum8/1
  Gain/1 -> Scope/5, Sum1/5
  Gain1/1 -> Scope/4, Sum1/4
  integralTerm/1(Out1) -> Transport Delay/1
  Sum/1 -> integralTerm/2(inputDiff)
  realInput/1 -> Integrator1/3, Sum/2
  Transport Delay/1 -> Scope/1, Sum1/1
  leaderChange/1 -> integralTerm/3(leaderChange)
  Demux/1 -> Saturation1/1  "eh"
  Kd/1 -> Scope/3, Sum1/3
  Demux/2 -> Kd/1  "ev"
  Saturation1/1 -> Kp/1, integralTerm/1(eh)
  errors/1 -> Demux/1
  Integrator1/1 -> Sum8/2
  Saturation/1 -> Integrator1/1
  Sum8/1 -> Gain3/1
  Gain3/1 -> Saturation/1
  Kp/1 -> Scope/2, Sum1/2
  inRange/1 -> integralTerm/Enable, Integrator1/2

== system CACC/F/Regular Vehicle Following/Velocity Control ==
  ev : Inport
  ea : Inport  Port=2
  realInput : Inport  Port=3
  Abs : Abs
  Compare To Constant : simulink/Logic and Bit Operations/Compare To Constant  relop=<=  const=0.2  OutDataTypeStr=boolean
  Constant : Constant  Value=.1
  Gain : Gain  Gain=velKd
  Scope : Scope  NumInputPorts=4
  Sum : Sum  Inputs=++|
  Sum1 : Sum  Inputs=|-+
  Sum3 : Sum  Inputs=+++
  Transport Delay : TransportDelay  DelayTime=0.1
  integral term : Subsystem
  velKp : Gain  Gain=velKp
  u : Outport  VectorParamsAs1DForOutWhenUnconnected=off
  wires:
  Transport Delay/1 -> Sum1/2
  Compare To Constant/1 -> integral term/Enable
  integral term/1(Out1) -> Sum3/1, Scope/1
  Abs/1 -> Compare To Constant/1
  Sum1/1 -> Abs/1
  ev/1 -> velKp/1, integral term/1(ev)
  velKp/1 -> Scope/2, Sum3/2
  Sum3/1 -> Sum/2, Scope/4, Transport Delay/1
  realInput/1 -> Sum1/1
  ea/1 -> Gain/1
  Gain/1 -> Scope/3, Sum3/3
  Constant/1 -> Sum/1
  Sum/1 -> u/1

== system CACC/F/Regular Vehicle Following/Velocity Error ==
  ego : Inport
  velRef : Inport  Port=2
  inRange : Inport  Port=3
  Bus Selector : BusSelector  OutputSignals=Xdot,xddot
  Gain : Gain  Gain=-1
  Gain3 : Gain  Gain=velFilterGain
  Integrator1 : Integrator  ExternalReset=rising  InitialCondition=vx0
  Saturation : Saturate  UpperLimit=maxComfAccel  LowerLimit=minComfAccel
  Sum : Sum  Inputs=+-|
  Sum8 : Sum  Inputs=|+-
  ev : Outport
  ea : Outport  Port=2
  wires:
  Sum8/1 -> Gain3/1
  Gain3/1 -> Saturation/1
  Saturation/1 -> Integrator1/1
  velRef/1 -> Sum8/1
  Integrator1/1 -> Sum/1, Sum8/2
  ego/1 -> Bus Selector/1
  Bus Selector/1 -> Sum/2  "<Xdot>"
  Bus Selector/2 -> Gain/1  "<xddot>"
  Sum/1 -> ev/1
  Gain/1 -> ea/1
  inRange/1 -> Integrator1/2

== system CACC/F/Regular Vehicle Following/switch free flow ==
  errors : Inport
  errorsDot : Inport  Port=2
  gap : Inport  Port=3
  h : Inport  Port=4
  d0 : Inport  Port=5
  vRef : Inport  Port=6
  Demux1 : Demux  Outputs=2
  Gain1 : Gain
  MATLAB Function : MATLAB Function  TreatAsAtomicUnit=on
  Relay : Relay  OnSwitchValue=1  OffSwitchValue=-1
  Scope : Scope  NumInputPorts=2
  Selector : Selector  InputPortWidth=2  IndexOptions=Index vector (dialog)  Indices=[2]  OutputSizes=1
  Sum2 : Sum  Inputs=-+
  inRange : Outport  VectorParamsAs1DForOutWhenUnconnected=off
  wires:
  Demux1/2 -> MATLAB Function/6(ea)
  Demux1/1 -> MATLAB Function/5(ehDot)
  errorsDot/1 -> Demux1/1
  MATLAB Function/1(maxGap) -> Sum2/2, Scope/2
  Gain1/1 -> MATLAB Function/1(h)
  Relay/1 -> inRange/1
  Selector/1 -> MATLAB Function/4(ev)
  Sum2/1 -> Relay/1
  gap/1 -> Sum2/1, Scope/1
  errors/1 -> Selector/1
  h/1 -> Gain1/1
  vRef/1 -> MATLAB Function/3(vRef)
  d0/1 -> MATLAB Function/2(d0)

== system CACC/F/findLeader/Subsystem ==
  ego : Inport
  all : Inport  Port=2
  Enable : EnablePort
  MATLAB Function : MATLAB Function  TreatAsAtomicUnit=on
  idx : Outport  InitialOutput=1  VectorParamsAs1DForOutWhenUnconnected=off
  wires:
  ego/1 -> MATLAB Function/1(ego)
  MATLAB Function/1(leaderIdx) -> idx/1
  all/1 -> MATLAB Function/2(allVehicles)

== system CACC/F/findLeader/farAwayVeh ==
  ego : Inport  OutDataTypeStr=Bus: vehStatesBus
  Bus Assignment : BusAssignment  AssignedSignals=X
  Bus Selector : BusSelector  OutputSignals=X
  Constant : Constant  Value=1000
  Sum : Sum  Inputs=|++
  Out1 : Outport  OutDataTypeStr=Bus: vehStatesBus  VectorParamsAs1DForOutWhenUnconnected=off
  wires:
  Sum/1 -> Bus Assignment/2  "X"
  Bus Selector/1 -> Sum/1  "<X>"
  Bus Assignment/1 -> Out1/1
  Constant/1 -> Sum/2
  ego/1 -> Bus Selector/1, Bus Assignment/1

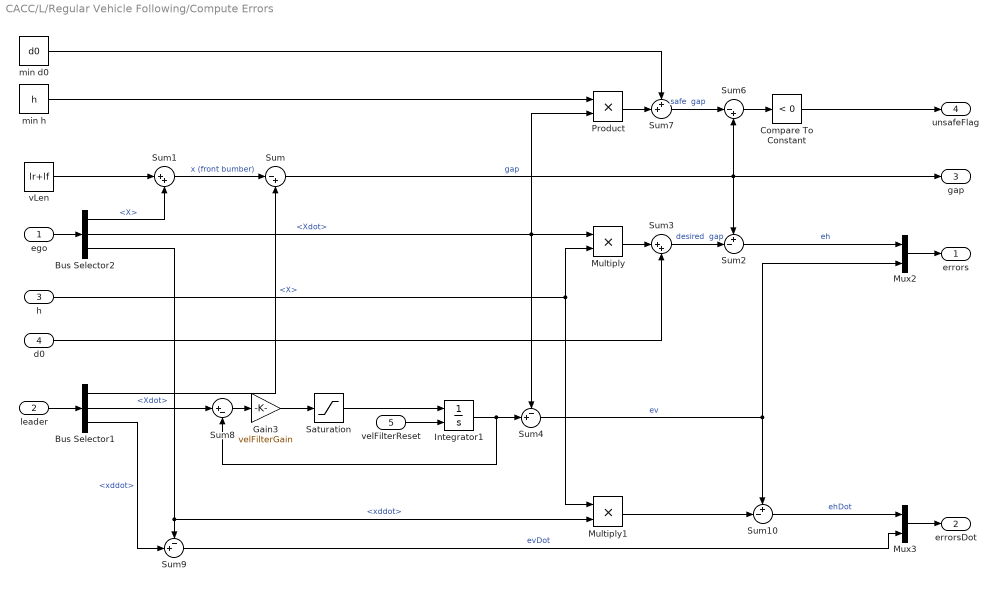
== system CACC/L/Regular Vehicle Following/Compute Errors ==
  ego : Inport
  leader : Inport  Port=2
  h : Inport  Port=3
  d0 : Inport  Port=4
  velFilterReset : Inport  Port=5
  Bus Selector1 : BusSelector  OutputSignals=X,Xdot,xddot
  Bus Selector2 : BusSelector  OutputSignals=X,Xdot,xddot
  Compare To Constant : simulink/Logic and Bit Operations/Compare To Constant  relop=<  const=0  OutDataTypeStr=boolean
  Gain3 : Gain  Gain=velFilterGain
  Integrator1 : Integrator  ExternalReset=rising  InitialCondition=vx0
  Multiply : Product
  Multiply1 : Product
  Mux2 : Mux  Inputs=2
  Mux3 : Mux  Inputs=2
  Product : Product
  Saturation : Saturate  UpperLimit=maxAcceleration  LowerLimit=minAcceleration
  Sum : Sum  Inputs=|-+
  Sum1 : Sum  Inputs=|++
  Sum10 : Sum  Inputs=+-|
  Sum2 : Sum  Inputs=+-|
  Sum3 : Sum  Inputs=|++
  Sum4 : Sum  Inputs=-+|
  Sum6 : Sum  Inputs=|-+
  Sum7 : Sum  Inputs=++|
  Sum8 : Sum  Inputs=|+-
  Sum9 : Sum  Inputs=-+|
  min d0 : Constant  Value=d0
  min h : Constant  Value=h
  vLen : Constant  Value=lr+lf
  errors : Outport  VectorParamsAs1DForOutWhenUnconnected=off
  errorsDot : Outport  Port=2
  "gap " : Outport  Port=3  VectorParamsAs1DForOutWhenUnconnected=off
  unsafeFlag : Outport  Port=4  VectorParamsAs1DForOutWhenUnconnected=off
  wires:
  leader/1 -> Bus Selector1/1
  ego/1 -> Bus Selector2/1
  Mux3/1 -> errorsDot/1
  Sum9/1 -> Mux3/2  "evDot"
  Sum10/1 -> Mux3/1  "ehDot"
  Multiply1/1 -> Sum10/2
  Bus Selector2/3 -> Multiply1/2, Sum9/1  "<xddot>"
  Bus Selector1/3 -> Sum9/2  "<xddot>"
  Sum8/1 -> Gain3/1
  Integrator1/1 -> Sum8/2, Sum4/2
  Saturation/1 -> Integrator1/1
  Gain3/1 -> Saturation/1
  Sum4/1 -> Sum10/1, Mux2/2  "ev"
  Bus Selector1/2 -> Sum8/1  "<Xdot>"
  h/1 -> Multiply1/1, Multiply/2
  Bus Selector2/1 -> Sum1/2  "<X>"
  Sum/1 -> Sum6/2, "gap "/1, Sum2/1  "gap"
  Multiply/1 -> Sum3/1
  min d0/1 -> Sum7/1
  vLen/1 -> Sum1/1
  d0/1 -> Sum3/2
  Bus Selector2/2 -> Product/2, Multiply/1, Sum4/1  "<Xdot>"
  Sum1/1 -> Sum/1  "x (front bumber)"
  Sum3/1 -> Sum2/2  "desired  gap"
  Product/1 -> Sum7/2
  Bus Selector1/1 -> Sum/2  "<X>"
  Sum2/1 -> Mux2/1  "eh"
  Compare To Constant/1 -> unsafeFlag/1
  min h/1 -> Product/1
  Sum7/1 -> Sum6/1  "safe  gap"
  Sum6/1 -> Compare To Constant/1
  velFilterReset/1 -> Integrator1/2
  Mux2/1 -> errors/1

== system CACC/L/Regular Vehicle Following/Define Desired Distance ==
  extraSpaceFlag : Inport
  Constant : Constant  Value=h
  Constant1 : Constant  Value=d0
  Constant2 : Constant  Value=hLC
  Constant3 : Constant  Value=d0LC
  Demux : Demux  Outputs=2
  Integrator : Integrator  InitialCondition=[h d0]
  Mux : Mux  Inputs=2
  Mux1 : Mux  Inputs=2
  Saturation1 : Saturate  UpperLimit=hFilterSaturation  LowerLimit=-hFilterSaturation
  Sum5 : Sum  Inputs=|+-
  Switch : Switch  Criteria=u2 > Threshold
  hFilterGain : Gain  Gain=hFilterGain
  h : Outport
  d0 : Outport  Port=2
  wires:
  Demux/2 -> d0/1
  Demux/1 -> h/1
  Integrator/1 -> Sum5/2, Demux/1
  Saturation1/1 -> Integrator/1
  extraSpaceFlag/1 -> Switch/2
  Constant1/1 -> Mux/2
  Constant3/1 -> Mux1/2
  Switch/1 -> Sum5/1
  Mux1/1 -> Switch/1
  Sum5/1 -> hFilterGain/1
  Constant2/1 -> Mux1/1
  hFilterGain/1 -> Saturation1/1
  Constant/1 -> Mux/1
  Mux/1 -> Switch/3

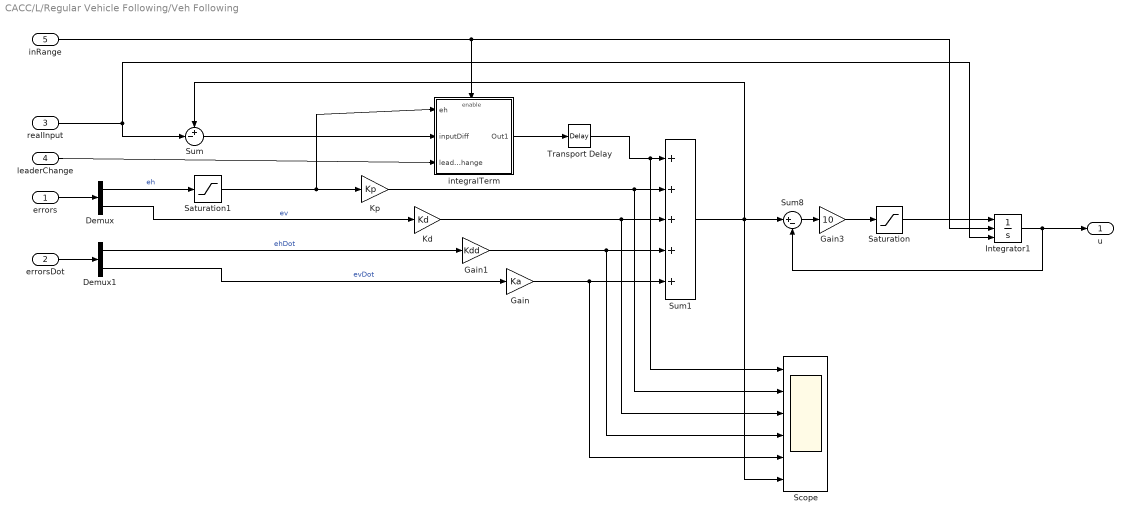
== system CACC/L/Regular Vehicle Following/Veh Following ==
  errors : Inport
  errorsDot : Inport  Port=2
  realInput : Inport  Port=3
  leaderChange : Inport  Port=4
  inRange : Inport  Port=5
  Demux : Demux  Outputs=2
  Demux1 : Demux  Outputs=2
  Gain : Gain  Gain=Ka
  Gain1 : Gain  Gain=Kdd
  Gain3 : Gain  Gain=10
  Integrator1 : Integrator  ExternalReset=rising  InitialConditionSource=external  InitialCondition=vx0
  Kd : Gain  Gain=Kd
  Kp : Gain  Gain=Kp
  Saturation : Saturate  UpperLimit=inf  LowerLimit=minAcceleration
  Saturation1 : Saturate  UpperLimit=maxHeadwayError  LowerLimit=minHeadwayError
  Scope : Scope  NumInputPorts=6
  Sum : Sum  Inputs=+-|
  Sum1 : Sum  Inputs=+++++
  Sum8 : Sum  Inputs=|+-
  Transport Delay : TransportDelay  DelayTime=0.1
  integralTerm : Subsystem
  u : Outport  VectorParamsAs1DForOutWhenUnconnected=off
  wires:
  Demux1/2 -> Gain/1  "evDot"
  Demux1/1 -> Gain1/1  "ehDot"
  errorsDot/1 -> Demux1/1
  Sum1/1 -> Scope/6, Sum/1, Sum8/1
  Gain/1 -> Scope/5, Sum1/5
  Gain1/1 -> Scope/4, Sum1/4
  integralTerm/1(Out1) -> Transport Delay/1
  Sum/1 -> integralTerm/2(inputDiff)
  realInput/1 -> Integrator1/3, Sum/2
  Transport Delay/1 -> Scope/1, Sum1/1
  inRange/1 -> integralTerm/Enable, Integrator1/2
  leaderChange/1 -> integralTerm/3(leaderChange)
  Demux/1 -> Saturation1/1  "eh"
  Kd/1 -> Scope/3, Sum1/3
  Demux/2 -> Kd/1  "ev"
  Saturation1/1 -> Kp/1, integralTerm/1(eh)
  errors/1 -> Demux/1
  Integrator1/1 -> Sum8/2, u/1
  Saturation/1 -> Integrator1/1
  Sum8/1 -> Gain3/1
  Gain3/1 -> Saturation/1
  Kp/1 -> Scope/2, Sum1/2

== system CACC/L/Regular Vehicle Following/Velocity Control ==
  ev : Inport
  ea : Inport  Port=2
  realInput : Inport  Port=3
  Abs : Abs
  Compare To Constant : simulink/Logic and Bit Operations/Compare To Constant  relop=<=  const=0.5  OutDataTypeStr=boolean
  Constant : Constant  Value=.1
  Gain : Gain  Gain=velKd
  Scope : Scope  NumInputPorts=4
  Sum : Sum  Inputs=++|
  Sum1 : Sum  Inputs=|-+
  Sum3 : Sum  Inputs=+++
  Transport Delay : TransportDelay  DelayTime=0.1
  integral term : Subsystem
  velKp : Gain  Gain=velKp
  u : Outport  VectorParamsAs1DForOutWhenUnconnected=off
  wires:
  Transport Delay/1 -> Sum1/2
  Compare To Constant/1 -> integral term/Enable
  integral term/1(Out1) -> Sum3/1, Scope/1
  Abs/1 -> Compare To Constant/1
  Sum1/1 -> Abs/1
  ev/1 -> velKp/1, integral term/1(ev)
  velKp/1 -> Scope/2, Sum3/2
  Sum3/1 -> Sum/2, Scope/4, Transport Delay/1
  realInput/1 -> Sum1/1
  ea/1 -> Gain/1
  Gain/1 -> Scope/3, Sum3/3
  Constant/1 -> Sum/1
  Sum/1 -> u/1

== system CACC/L/Regular Vehicle Following/Velocity Error ==
  ego : Inport
  velRef : Inport  Port=2
  inRange : Inport  Port=3
  Bus Selector : BusSelector  OutputSignals=Xdot,xddot
  Gain : Gain  Gain=-1
  Gain3 : Gain  Gain=velFilterGain
  Integrator1 : Integrator  ExternalReset=rising  InitialCondition=vx0
  Saturation : Saturate  UpperLimit=maxComfAccel  LowerLimit=minComfAccel
  Sum : Sum  Inputs=+-|
  Sum8 : Sum  Inputs=|+-
  ev : Outport
  ea : Outport  Port=2
  wires:
  Sum8/1 -> Gain3/1
  Gain3/1 -> Saturation/1
  Saturation/1 -> Integrator1/1
  velRef/1 -> Sum8/1
  Integrator1/1 -> Sum/1, Sum8/2
  ego/1 -> Bus Selector/1
  Bus Selector/1 -> Sum/2  "<Xdot>"
  Bus Selector/2 -> Gain/1  "<xddot>"
  Sum/1 -> ev/1
  Gain/1 -> ea/1
  inRange/1 -> Integrator1/2

== system CACC/L/Regular Vehicle Following/switch ==
  errors : Inport
  errorsDot : Inport  Port=2
  gap : Inport  Port=3
  h : Inport  Port=4
  d0 : Inport  Port=5
  vRef : Inport  Port=6
  Compare To Constant : simulink/Logic and Bit Operations/Compare To Constant  relop=<=  const=0  OutDataTypeStr=boolean
  Demux1 : Demux  Outputs=2
  Gain1 : Gain
  MATLAB Function : MATLAB Function  TreatAsAtomicUnit=on
  Scope : Scope  NumInputPorts=2
  Selector : Selector  InputPortWidth=2  IndexOptions=Index vector (dialog)  Indices=[2]  OutputSizes=1
  Sum2 : Sum  Inputs=+-
  inRange : Outport  VectorParamsAs1DForOutWhenUnconnected=off
  wires:
  Demux1/2 -> MATLAB Function/6(ea)
  Demux1/1 -> MATLAB Function/5(ehDot)
  errorsDot/1 -> Demux1/1
  MATLAB Function/1(maxGap) -> Sum2/2, Scope/2
  Gain1/1 -> MATLAB Function/1(h)
  Compare To Constant/1 -> inRange/1
  Selector/1 -> MATLAB Function/4(ev)
  Sum2/1 -> Compare To Constant/1
  gap/1 -> Sum2/1, Scope/1
  errors/1 -> Selector/1
  h/1 -> Gain1/1
  vRef/1 -> MATLAB Function/3(vRef)
  d0/1 -> MATLAB Function/2(d0)

== system CACC/L/findLeader/Subsystem ==
  ego : Inport
  all : Inport  Port=2
  Enable : EnablePort
  MATLAB Function : MATLAB Function  TreatAsAtomicUnit=on
  idx : Outport  InitialOutput=1  VectorParamsAs1DForOutWhenUnconnected=off
  wires:
  ego/1 -> MATLAB Function/1(ego)
  MATLAB Function/1(leaderIdx) -> idx/1
  all/1 -> MATLAB Function/2(allVehicles)

== system CACC/L/findLeader/farAwayVeh ==
  ego : Inport  OutDataTypeStr=Bus: vehStatesBus
  Bus Assignment : BusAssignment  AssignedSignals=X
  Bus Selector : BusSelector  OutputSignals=X
  Constant : Constant  Value=1000
  Sum : Sum  Inputs=|++
  Out1 : Outport  OutDataTypeStr=Bus: vehStatesBus  VectorParamsAs1DForOutWhenUnconnected=off
  wires:
  Sum/1 -> Bus Assignment/2  "X"
  Bus Selector/1 -> Sum/1  "<X>"
  Bus Assignment/1 -> Out1/1
  Constant/1 -> Sum/2
  ego/1 -> Bus Selector/1, Bus Assignment/1

== system CACC/F/Regular Vehicle Following/Veh Following/integralTerm ==
  eh : Inport
  inputDiff : Inport  Port=2
  leaderChange : Inport  Port=3
  Enable : EnablePort  ShowOutputPort=on
  Anti-windup gain : Gain  Gain=sqrt(Ki/Kd)
  Integrator : Integrator  ExternalReset=either
  Ki : Gain  Gain=Ki
  Scope : Scope  NumInputPorts=2
  Sum5 : Sum  Inputs=-+|
  XOR : Logic  Operator=XOR  IconShape=distinctive  AllPortsSameDT=off  OutDataTypeStr=boolean
  Out1 : Outport  OutputWhenDisabled=reset  InitialOutput=0  VectorParamsAs1DForOutWhenUnconnected=off
  wires:
  inputDiff/1 -> Anti-windup gain/1
  Anti-windup gain/1 -> Scope/1, Sum5/1
  Ki/1 -> Sum5/2
  Sum5/1 -> Scope/2, Integrator/1
  Enable/1 -> XOR/2
  leaderChange/1 -> XOR/1
  XOR/1 -> Integrator/2
  Integrator/1 -> Out1/1
  eh/1 -> Ki/1

== system CACC/F/Regular Vehicle Following/Velocity Control/integral term ==
  ev : Inport
  Enable : EnablePort  StatesWhenEnabling=reset
  Integrator2 : Integrator
  velKi : Gain  Gain=velKi
  Out1 : Outport  OutputWhenDisabled=reset  InitialOutput=0
  wires:
  ev/1 -> velKi/1
  Integrator2/1 -> Out1/1
  velKi/1 -> Integrator2/1

== system CACC/L/Regular Vehicle Following/Veh Following/integralTerm ==
  eh : Inport
  inputDiff : Inport  Port=2
  leaderChange : Inport  Port=3
  Enable : EnablePort  ShowOutputPort=on
  Anti-windup gain : Gain  Gain=sqrt(Ki/Kd)
  Integrator : Integrator  ExternalReset=either
  Ki : Gain  Gain=Ki
  Sum5 : Sum  Inputs=-+|
  XOR : Logic  Operator=XOR  IconShape=distinctive  AllPortsSameDT=off  OutDataTypeStr=boolean
  Out1 : Outport  OutputWhenDisabled=reset  InitialOutput=0  VectorParamsAs1DForOutWhenUnconnected=off
  wires:
  inputDiff/1 -> Anti-windup gain/1
  Anti-windup gain/1 -> Sum5/1
  Ki/1 -> Sum5/2
  Sum5/1 -> Integrator/1
  Enable/1 -> XOR/2
  leaderChange/1 -> XOR/1
  XOR/1 -> Integrator/2
  Integrator/1 -> Out1/1
  eh/1 -> Ki/1

== system CACC/L/Regular Vehicle Following/Velocity Control/integral term ==
  ev : Inport
  Enable : EnablePort  StatesWhenEnabling=reset
  Integrator2 : Integrator
  velKi : Gain  Gain=velKi
  Out1 : Outport  OutputWhenDisabled=reset  InitialOutput=0
  wires:
  ev/1 -> velKi/1
  Integrator2/1 -> Out1/1
  velKi/1 -> Integrator2/1

== matlab function CACC/F/findLeader/Subsystem/MATLAB Function ==
  data: ego input Bus: vehStatesBus; allVehicles input; leaderIdx output
function leaderIdx  = findLeader(ego, allVehicles)

nv = length(allVehicles);

leaderIdx = nv+1;

farAwayVehicle.X = ego.X + 10^4;
farAwayVehicle.Y = ego.Y;
farAwayVehicle.Xdot = ego.Xdot;
farAwayVehicle.u = 0;

leader = farAwayVehicle;
% For non lane changing vehicles, the leader is whoever is longitudinally
% closer and with any part of the body in the same lane.
% 1.8m (half lane) + 0.9m (half veh width)
for n = 1:nv
    if allVehicles(n).X>ego.X
        if abs(allVehicles(n).Y - ego.Y)<=2.7 && allVehicles(n).X<leader.X
            leaderIdx = n;
        end
    end
end

== matlab function CACC/L/Regular Vehicle Following/switch/MATLAB Function ==
  data: h input; maxGap output; d0 input; vRef input; ev input; ehDot input; ea input; Kp parameter; Kd parameter; Ka parameter; Kdd parameter
function maxGap = followingGapThreshold(h, d0, vRef, ev, ehDot, ea, Kp, Kd, Ka, Kdd)

maxGap = h*vRef + d0 - 1/Kp*(Kd*ev + Kdd*ehDot + Ka*ea);

== matlab function CACC/F/Regular Vehicle Following/switch free flow/MATLAB Function ==
  data: h input; maxGap output; d0 input; vRef input; ev input; ehDot input; ea input; Kp parameter; Kd parameter; Ka parameter; Kdd parameter
function maxGap = followingGapThreshold(h, d0, vRef, ev, ehDot, ea, Kp, Kd, Ka, Kdd)

maxGap = h*vRef + d0 - 1/Kp*(Kd*ev + Kdd*ehDot + Ka*ea);

== matlab function CACC/L/findLeader/Subsystem/MATLAB Function ==
  data: ego input Bus: vehStatesBus; allVehicles input; leaderIdx output
function leaderIdx  = findLeader(ego, allVehicles)

nv = length(allVehicles);

leaderIdx = nv+1;

farAwayVehicle.X = ego.X + 10^4;
farAwayVehicle.Y = ego.Y;
farAwayVehicle.Xdot = ego.Xdot;
farAwayVehicle.u = 0;

leader = farAwayVehicle;
% For non lane changing vehicles, the leader is whoever is longitudinally
% closer and with any part of the body in the same lane.
% 1.8m (half lane) + 0.9m (half veh width)
for n = 1:nv
    if allVehicles(n).X>ego.X
        if abs(allVehicles(n).Y - ego.Y)<=2.7 && allVehicles(n).X<leader.X
            leaderIdx = n;
        end
    end
end
